simulink subsystem "IMU"  (R2023a)
settings: Solver=VariableStepAuto  StartTime=0.0  StopTime=10.0  RelTol=1e-3
settings Model: Creator=jonvargas  LastModifiedBy=jonvargas

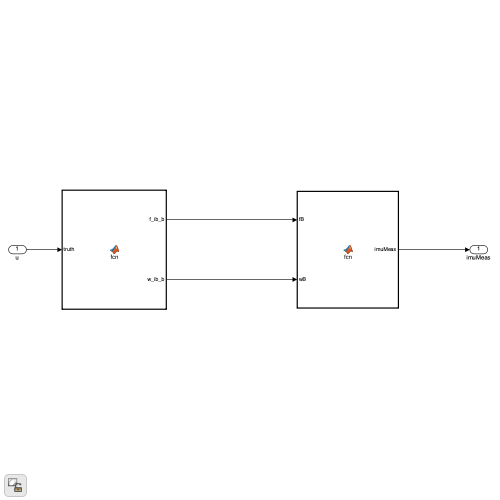
[thumbnail: Simulink's stored preview of the top-level diagram]
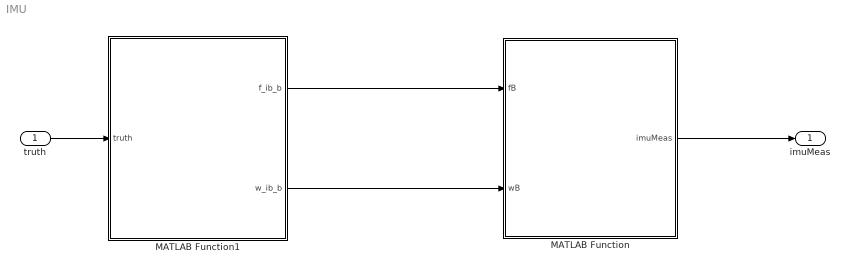
== system IMU ==
  truth : Inport
  MATLAB Function : MATLAB Function  TreatAsAtomicUnit=on
  MATLAB Function1 : MATLAB Function  TreatAsAtomicUnit=on
  imuMeas : Outport
  wires:
  MATLAB Function/1(imuMeas) -> imuMeas/1
  truth/1 -> MATLAB Function1/1(truth)
  MATLAB Function1/1(f_ib_b) -> MATLAB Function/1(fB)
  MATLAB Function1/2(w_ib_b) -> MATLAB Function/2(wB)

== matlab function IMU/MATLAB Function ==
  data: fB input; imuMeas output; wB input; params parameter
function imuMeas =  fcn(fB,wB,params)


imuMeas = imu_sensor(fB,wB,params)

== matlab function IMU/MATLAB Function1 ==
  data: truth input; f_ib_b output; w_ib_b output; params parameter
function [f_ib_b, w_ib_b]= fcn(truth,params)

[f_ib_b, w_ib_b] = imuData(truth,params);
